simulink model "TestMultiPath"  (R2022b)
settings: Solver=VariableStepAuto  StartTime=0.0  StopTime=10.0  RelTol=1e-3
settings Model: PacingRate=0.050000  Creator=ADMIN  LastModifiedBy=ADMIN

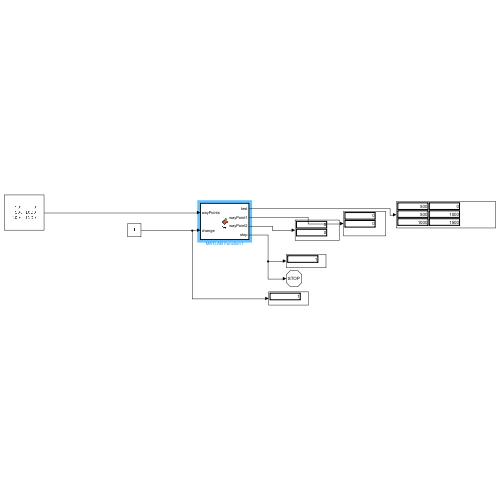
[thumbnail: Simulink's stored preview of the top-level diagram]
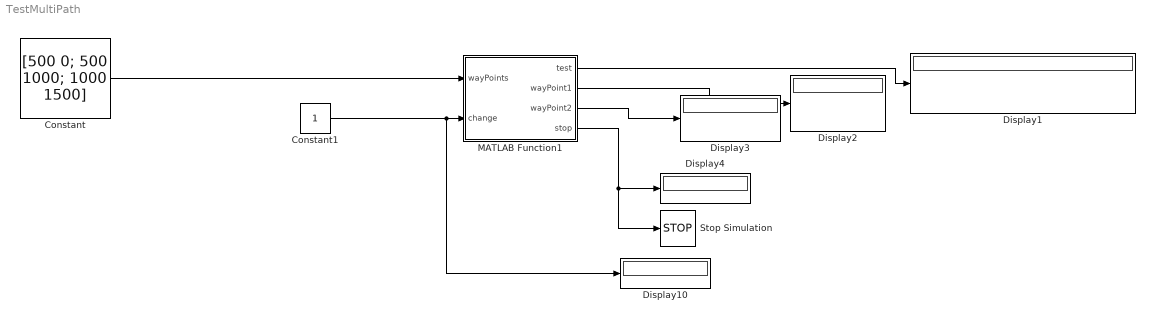
== system TestMultiPath ==
  Constant : Constant  Value=[500 0; 500 1000; 1000 1500]
  Constant1 : Constant
  Display{1..4,10} (5 alike) : Display
  MATLAB Function1 : MATLAB Function  TreatAsAtomicUnit=on
  Stop Simulation : Stop
  wires:
  Constant/1 -> MATLAB Function1/1(wayPoints)
  Constant1/1 -> Display10/1, MATLAB Function1/2(change)
  MATLAB Function1/1(test) -> Display1/1
  MATLAB Function1/2(wayPoint1) -> Display2/1
  MATLAB Function1/3(wayPoint2) -> Display3/1
  MATLAB Function1/4(stop) -> Display4/1, Stop Simulation/1

== matlab function TestMultiPath/MATLAB Function1 ==
  data: test output; wayPoint1 output; wayPoint2 output; wayPoints input; change input; stop output
function [test, wayPoint1, wayPoint2, stop] = fcn(wayPoints, change)
test = wayPoints;
stop = 0;
wayPoint1 = [0;0];
wayPoint2 = [0;0];
persistent current
if isempty(current)
   current = 0;
end

if isempty(change)
   change = 1;
end

persistent s
s = size(wayPoints,1);
if change
   current = current + 1
   if current == s
      stop = 1
      disp('exceed')
      return
   else
      wayPoint1 = wayPoints(current,:)'
      wayPoint2 = wayPoints(current+1,:)'
   end
else
   wayPoint1 = wayPoints(current,:)'
   wayPoint2 = wayPoints(current+1,:)'
end
